simulink model "double_integrator"  (R2014b)
settings: Solver=FixedStepDiscrete  SolverMode=SingleTasking  StartTime=0.0  StopTime=Tsim  FixedStep=Ts  RelTol=1e-3
InitFcn:
  | config
libraries: simulink x1
settings Model: CovMetricSettings=dwe  CovHtmlReporting=off  covSaveCumulativeToWorkspaceVar=off  CovSaveSingleToWorkspaceVar=off  CovExternalEMLEnable=on  CovSFcnEnable=on  Creator=mnade  LastModifiedBy=nina
settings DataIOCC: LimitDataPoints=off  SaveFormat=StructureWithTime
settings DebuggingCC: SolverPrmCheckMsg=none  FrameProcessingCompatibilityMsg=error  SFUnexpectedBacktrackingDiag=error  SFNoUnconditionalDefaultTransitionDiag=error
settings HardwareCC: ProdBitPerPointer=64  ProdLargestAtomicFloat=Float  ProdIntDivRoundTo=Zero  ProdEndianess=LittleEndian  ProdHWDeviceType=Specified
settings ModelReferenceCC: PropagateSignalLabelsOutOfModel=on
settings GRTTargetCC: TargetLangStandard=C99 (ISO)  GeneratePreprocessorConditionals=Use local settings

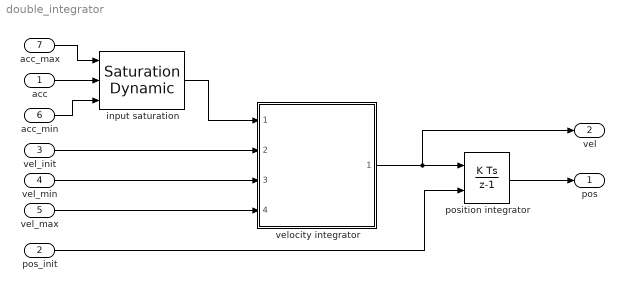
== system double_integrator ==
  acc : Inport
  pos_init : Inport  Port=2
  vel_init : Inport  Port=3
  vel_min : Inport  Port=4
  vel_max : Inport  Port=5
  acc_min : Inport  Port=6
  acc_max : Inport  Port=7
  input saturation : simulink/Discontinuities/Saturation Dynamic  OutMin=[]  OutMax=[]  OutDataTypeStr=Inherit: Same as second input  OutDataType=fixdt(1, 16)  OutScaling=2^-10  DoSatur=off
  position integrator : DiscreteIntegrator  InitialConditionSource=external  InitialConditionSetting=State (most efficient)  SampleTime=-1
  velocity integrator : ModelReference  ModelNameDialog=integrator_with_state_boundaries.slx  SimulationMode=Normal  ModelReferenceVersion=1.16  CopyOfModelName=integrator_with_state_boundaries.slx  DefaultDataLogging=on
  pos : Outport
  vel : Outport  Port=2
  wires:
  velocity integrator/1 -> vel/1, position integrator/1
  position integrator/1 -> pos/1
  vel_init/1 -> velocity integrator/2
  pos_init/1 -> position integrator/2
  acc/1 -> input saturation/2
  input saturation/1 -> velocity integrator/1
  acc_max/1 -> input saturation/1
  acc_min/1 -> input saturation/3
  vel_min/1 -> velocity integrator/3
  vel_max/1 -> velocity integrator/4
